simulink model "w31_v6"  (Simulink 7.9)
settings: Solver=FixedStepDiscrete  StartTime=0.0  StopTime=inf  FixedStep=0.01  RelTol=1e-3
undefined symbols (not defined in the file): DiscIntNeverNeededParam, magnitude
libraries: canmsglib x24, cansrvlib x22, simulink x12, iohwablib x5, legionoslib x3, ccpsrvlib x2, memsrvlib x1, tgttoollib x1, udssrvlib x1, wdgmlib x1
(part 2 of 5)

== system w31_v6/Logic_And_Algorithm/No_Signal_Emg_Judge ==
  Chassis_Signal : Inport
  Remote_Signal : Inport  Port=2
  Hardware_Signal : Inport  Port=3
  iECU_Signal : Inport  Port=4
  Bus Creator : BusCreator  Inputs=1
  Bus Creator1 : BusCreator  Inputs=1
  Bus Selector : BusSelector  OutputSignals=DBSF_Receive.DBSF_Status_NoRxMsg
  Bus Selector1 : BusSelector  OutputSignals=Remote_Analog.Remote_Analog_Status,Remote_IO.Remote_IO_Status
  Bus Selector2 : BusSelector  OutputSignals=Eme_Stop_Cmd,Front_Touch_Switch,Rear_Touch_Switch
  Bus Selector3 : BusSelector  OutputSignals=iECU_Status
  Logical Operator : Logic  Operator=OR  Inputs=6  AllPortsSameDT=off  OutDataTypeStr=boolean
  Logical Operator1 : Logic  Operator=OR  AllPortsSameDT=off  OutDataTypeStr=boolean
  No_Remote_CAN_Msg_Or_Emg_Button : Outport
  No_iECU_CAN_Msg_Or_Emg_Button : Outport  Port=2
  wires:
  Chassis_Signal/1 -> Bus Selector/1
  Remote_Signal/1 -> Bus Selector1/1
  Hardware_Signal/1 -> Bus Selector2/1
  iECU_Signal/1 -> Bus Selector3/1
  Bus Selector/1 -> Logical Operator/1  "<DBSF_Status_NoRxMsg>"
  Bus Selector1/1 -> Logical Operator/3  "<Remote_Analog_Status>"
  Bus Selector1/2 -> Logical Operator/4  "<Remote_IO_Status>"
  Logical Operator/1 -> Bus Creator/1, Logical Operator1/1  "No_Remote_CAN_Msg_Or_Emg_Button"
  Logical Operator1/1 -> Bus Creator1/1  "No_iECU_CAN_Msg_Or_Emg_Button"
  Bus Selector3/1 -> Logical Operator1/2  "<iECU_Status>"
  Bus Creator/1 -> No_Remote_CAN_Msg_Or_Emg_Button/1  "No_Remote_CAN_Msg_Or_Emg_Button"
  Bus Creator1/1 -> No_iECU_CAN_Msg_Or_Emg_Button/1
  Bus Selector2/1 -> Logical Operator/2  "<Eme_Stop_Cmd>"
  Bus Selector2/2 -> Logical Operator/5  "<Front_Touch_Switch>"
  Bus Selector2/3 -> Logical Operator/6  "<Rear_Touch_Switch>"

== system w31_v6/Logic_And_Algorithm/Remote_mode_with_control_0 ==
  note: 驱动控制算法，等待填充分布式控制算法
  Chassis_CAN_input : Inport
  Sensor_CAN_input : Inport  Port=2
  Remote_CAN_input : Inport  Port=3
  Hardware_input : Inport  Port=4
  No_Remote_CAN_Msg_Or_Emg_Button : Inport  Port=5
  Action Port : ActionPort  ActionType=case
  Brake_calculation : Subsystem
  Bus Creator : BusCreator
  Bus Creator1 : BusCreator  Inputs=6
  Bus Creator2 : BusCreator  Inputs=2
  Power_calculation : Subsystem
  Signal_Input : Subsystem
  Steering_calculation : Subsystem
  Power_cal_to_CANBus : Outport
  Steering_cal_to_CANBus : Outport  Port=2
  Brake_to_CANBus : Outport  Port=3
  wires:
  Bus Creator/1 -> Power_cal_to_CANBus/1
  Chassis_CAN_input/1 -> Signal_Input/1(Chassis_CAN_input)
  Sensor_CAN_input/1 -> Signal_Input/2(Sensor_CAN_input)
  Remote_CAN_input/1 -> Signal_Input/3(Remote_CAN_input)
  Hardware_input/1 -> Signal_Input/4(Hardware_input)
  Bus Creator1/1 -> Steering_cal_to_CANBus/1
  Steering_calculation/1(F_Steering_Angle) -> Bus Creator1/1
  Steering_calculation/2(R_Steering_Angle) -> Bus Creator1/2
  Steering_calculation/3(F_Steering_Work_Mode) -> Bus Creator1/3
  Steering_calculation/4(R_Steering_Work_Mode) -> Bus Creator1/4
  Steering_calculation/5(F_Steering_Angle_Rate) -> Bus Creator1/5
  Steering_calculation/6(R_Steering_Angle_Rate) -> Bus Creator1/6
  No_Remote_CAN_Msg_Or_Emg_Button/1 -> Signal_Input/5(No_Remote_CAN_Msg_Or_Emg_Button)
  Brake_calculation/1(Break_Req) -> Bus Creator2/1  "Break_Req"
  Brake_calculation/2(Remote_EPB_Req) -> Bus Creator2/2  "Remote_EPB_Req"
  Bus Creator2/1 -> Brake_to_CANBus/1
  Power_calculation/1(Power_FL) -> Bus Creator/1
  Power_calculation/2(Power_FR) -> Bus Creator/2
  Power_calculation/3(Power_RL) -> Bus Creator/3
  Power_calculation/4(Power_RR) -> Bus Creator/4

== system w31_v6/Logic_And_Algorithm/Remote_mode_with_control_2 ==
  note: 驱动控制算法，等待填充分布式控制算法
  Remote_CAN_input : Inport
  Hardware_input : Inport  Port=2
  No_Remote_CAN_Msg_Or_Emg_Button : Inport  Port=3
  Action Port : ActionPort  ActionType=case
  Brake_calculation : Subsystem
  Bus Creator : BusCreator
  Bus Creator1 : BusCreator  Inputs=6
  Bus Creator2 : BusCreator  Inputs=2
  Power_calculation : Subsystem
  Signal_Input : Subsystem
  Steering_calculation : Subsystem
  Steering_cal_to_CANBus : Outport
  Brake_to_CANBus : Outport  Port=2
  Power_cal_to_CANBus : Outport  Port=3
  wires:
  No_Remote_CAN_Msg_Or_Emg_Button/1 -> Signal_Input/3(No_Remote_CAN_Msg_Or_Emg_Button)
  Hardware_input/1 -> Signal_Input/2(Hardware_input)
  Remote_CAN_input/1 -> Signal_Input/1(Remote_CAN_input)
  Bus Creator2/1 -> Brake_to_CANBus/1
  Brake_calculation/2(Remote_EPB_Req) -> Bus Creator2/2  "Remote_EPB_Req"
  Brake_calculation/1(Break_Req) -> Bus Creator2/1  "Break_Req"
  Steering_calculation/6(R_Steering_Angle_Rate) -> Bus Creator1/6
  Steering_calculation/5(F_Steering_Angle_Rate) -> Bus Creator1/5
  Steering_calculation/4(R_Steering_Work_Mode) -> Bus Creator1/4
  Steering_calculation/3(F_Steering_Work_Mode) -> Bus Creator1/3
  Steering_calculation/2(R_Steering_Angle) -> Bus Creator1/2
  Steering_calculation/1(F_Steering_Angle) -> Bus Creator1/1
  Bus Creator1/1 -> Steering_cal_to_CANBus/1
  Bus Creator/1 -> Power_cal_to_CANBus/1
  Power_calculation/1(Power_FL) -> Bus Creator/1
  Power_calculation/2(Power_FR) -> Bus Creator/2
  Power_calculation/3(Power_RL) -> Bus Creator/3
  Power_calculation/4(Power_RR) -> Bus Creator/4

== system w31_v6/Logic_And_Algorithm/Slop_Cal ==
  IMU_Ax : Inport
  Trigonometric Function : Trigonometry  Operator=asin
  Slop : Outport
  wires:
  IMU_Ax/1 -> Trigonometric Function/1
  Trigonometric Function/1 -> Slop/1

== system w31_v6/Logic_And_Algorithm/drive_mode_judegment ==
  note: Remote请求为0，iECU请求为1的情况下，输出非0，进入自动驾驶状态，否则为遥控驾驶
  Remote_CANbus : Inport
  iECU_CANbus : Inport  Port=2
  Bus Selector : BusSelector  OutputSignals=Remote_IO.Remote_or_iECU_Mode_Switch,Remote_IO.Remote_Control_Speed_or_Torque
  Bus Selector1 : BusSelector  OutputSignals=iECU_Control_Flag
  Data Type Conversion3 : DataTypeConversion  OutDataTypeStr=uint8
  MATLAB Function : MATLAB Function  TreatAsAtomicUnit=on
  drive_mode : Outport
  wires:
  Remote_CANbus/1 -> Bus Selector/1
  iECU_CANbus/1 -> Bus Selector1/1
  Bus Selector/1 -> MATLAB Function/1(remote_or_iECU)  "<Remote_or_iECU_Mode_Switch>"
  Bus Selector/2 -> MATLAB Function/2(remote_speed_or_torque)  "<Remote_Control_Speed_or_Torque>"
  Bus Selector1/1 -> MATLAB Function/3(iECU_control_flag)  "<iECU_Control_Flag>"
  MATLAB Function/1(drive_mode) -> Data Type Conversion3/1
  Data Type Conversion3/1 -> drive_mode/1

== system w31_v6/Logic_And_Algorithm/iECU_mode_with_control ==
  note: 驱动控制算法，等待填充分布式控制算法
  Chassis_CAN_input : Inport
  Sensor_CAN_input : Inport  Port=2
  Remote_CAN_input : Inport  Port=3
  Hardware_input : Inport  Port=4
  iECU_CAN_input : Inport  Port=5
  No_iECU_CAN_Msg_Or_Emg_Button : Inport  Port=6
  Action Port : ActionPort  ActionType=default
  Brake_calculation : Subsystem
  Bus Creator : BusCreator  Inputs=2
  Bus Creator1 : BusCreator  Inputs=6
  Power_calculation : Subsystem
  Signal_Input : Subsystem
  Steering_calculation : Subsystem
  Power_cal_to_CANBus : Outport
  Steering_cal_to_CANBus : Outport  Port=2
  Brake_to_CANBus : Outport  Port=3
  wires:
  Chassis_CAN_input/1 -> Signal_Input/1(Chassis_CAN_input)
  Sensor_CAN_input/1 -> Signal_Input/2(Sensor_CAN_input)
  Remote_CAN_input/1 -> Signal_Input/3(Remote_CAN_input)
  Hardware_input/1 -> Signal_Input/4(Hardware_input)
  iECU_CAN_input/1 -> Signal_Input/5(iECU_CAN_input)
  Bus Creator/1 -> Power_cal_to_CANBus/1
  Power_calculation/2(Torque_to_Motor_CANBus) -> Bus Creator/2
  Bus Creator1/1 -> Steering_cal_to_CANBus/1
  Steering_calculation/1(F_Steering_Angle) -> Bus Creator1/1
  Steering_calculation/2(R_Steering_Angle) -> Bus Creator1/2
  Steering_calculation/3(F_Steering_Work_Mode) -> Bus Creator1/3
  Steering_calculation/4(R_Steering_Work_Mode) -> Bus Creator1/4
  Steering_calculation/5(F_Steering_Angle_Rate) -> Bus Creator1/5
  Steering_calculation/6(R_Steering_Angle_Rate) -> Bus Creator1/6
  Brake_calculation/1(Break_Req) -> Brake_to_CANBus/1  "Break_Req"
  No_iECU_CAN_Msg_Or_Emg_Button/1 -> Signal_Input/6(No_iECU_CAN_Msg_Or_Emg_Button)
  Power_calculation/1(Rotation_to_Motor_CANBus) -> Bus Creator/1

== system w31_v6/10ms_Signal_Output/SteerCAN_Out1/F ==
  Command_Angle : Inport
  Bitwise Operator : simulink/Logic and Bit Operations/Bitwise Operator  logicop=XOR  UseBitMask=off  NumInputPorts=7  BitMask=bin2dec('11011001')  BitMaskRealWorld=Stored Integer
  CAN Pack1 : canmsglib/CAN Pack  CANdbFile=E:\matlab_ws\2012_Matlab_Vcu\w_serial\w3\w32\dbc\w32_CAN1_500kbs_0421_v15.dbc  MsgList=VCU_EPSF_Control_Request  MsgName=VCU_EPSF_Control_Request  MsgIDType=Standard (11-bit identifier)  MsgIdentifier=1129  MsgLength=8  SignalInfo=High_VCU_Req_EPSF_Target_Angle$24$8$1$2$1$0$1$0$0$255$#Low_VCU_Req_EPSF_Target_Angle$32$8$1$2$1$0$1$0$0$255$#VCU_Control_EPSF_Reserved_1$8$8$1$2$1$0$1$0$0$255$#VCU_Control_EPSF_Reserved_2$16$8$1$2$1$0$1$0$0$255$#VCU_EPSF_CheckSum$56$8$1$2$1$0$1$0$0$255$#VCU_Request_EPSF_Angle_Calibrate$40$8$1$2$1$0$1$0$0$255$#VCU_Request_EPSF_Angle_Speed$48$8$1$2$1$0$1$0$20$250$#VCU_Request_EPSF_Control_Mode$0$8$1$2$1$0$1$0$0$255$#  NSignals=8  StartBits=str2num('[int32(24);int32(32);int32(8);int32(16);int32(56);int32(40);int32(48);int32(0)]')  SignalSizes=str2num('[int32(8);int32(8);int32(8);int32(8);int32(8);int32(8);int32(8);int32(8)]')  ByteOrders=str2num('[int32(1);int32(1);int32(1);int32(1);int32(1);int32(1);int32(1);int32(1)]')  DataTypes=str2num('[int32(2);int32(2);int32(2);int32(2);int32(2);int32(2);int32(2);int32(2)]')  MultiplexTypes=str2num('[int32(1);int32(1);int32(1);int32(1);int32(1);int32(1);int32(1);int32(1)]')  MultiplexValues=str2num('[double(0);double(0);double(0);double(0);double(0);double(0);double(0);double(0)]')  Factors=str2num('[double(1);double(1);double(1);double(1);double(1);double(1);double(1);double(1)]')  Offsets=str2num('[double(0);double(0);double(0);double(0);double(0);double(0);double(0);double(0)]')  Minimums=str2num('[double(0);double(0);double(0);double(0);double(0);double(0);double(20);double(0)]')  Maximums=str2num('[double(255);double(255);double(255);double(255);double(255);double(255);double(250);double(255)]')  Remote=off
      settings: DataFormat=CANdb specified signals
  CAN Transmit1 : cansrvlib/CAN Transmit  useModule=CAN1  messageID=hex2dec('469')  messageType=Standard (11-bit identifier)  msg_priority=255  messageID_Numeric=1129  ECU=V11P51_00E170701_01
  Subsystem : Subsystem
  eps_control_mode : Constant  Value=200  OutDataTypeStr=uint8  SampleTime=-1
  eps_reserve_1 : Constant  Value=0  OutDataTypeStr=uint8  SampleTime=-1
  eps_reserve_2 : Constant  Value=0  OutDataTypeStr=uint8  SampleTime=-1
  eps_reserve_3 : Constant  Value=32  OutDataTypeStr=uint8  SampleTime=-1
  eps_reserve_4 : Constant  Value=0  OutDataTypeStr=uint8  SampleTime=-1
  wires:
  CAN Pack1/1 -> CAN Transmit1/1
  Command_Angle/1 -> Subsystem/1(deserved_angle)
  eps_reserve_4/1 -> CAN Pack1/3, Bitwise Operator/2
  Subsystem/1(cmd_angle_high) -> CAN Pack1/1, Bitwise Operator/4
  Subsystem/2(cmd_angle_low) -> CAN Pack1/2, Bitwise Operator/5
  eps_reserve_1/1 -> CAN Pack1/4, Bitwise Operator/3
  eps_reserve_2/1 -> CAN Pack1/6, Bitwise Operator/6
  eps_control_mode/1 -> CAN Pack1/7, Bitwise Operator/7
  eps_reserve_3/1 -> CAN Pack1/8, Bitwise Operator/1
  Bitwise Operator/1 -> CAN Pack1/5

== system w31_v6/10ms_Signal_Output/SteerCAN_Out1/R ==
  Command_Angle : Inport
  Bitwise Operator : simulink/Logic and Bit Operations/Bitwise Operator  logicop=XOR  UseBitMask=off  NumInputPorts=7  BitMask=bin2dec('11011001')  BitMaskRealWorld=Stored Integer
  CAN Pack1 : canmsglib/CAN Pack  CANdbFile=E:\matlab_ws\2012_Matlab_Vcu\w_serial\w3\w32\dbc\w32_CAN1_500kbs_0421_v15.dbc  MsgList=VCU_EPSR_Control_Request  MsgName=VCU_EPSR_Control_Request  MsgIDType=Standard (11-bit identifier)  MsgIdentifier=257  MsgLength=8  SignalInfo=High_VCU_Req_EPSR_Target_Angle$24$8$1$2$1$0$1$0$0$255$#Low_VCU_Req_EPSR_Target_Angle$32$8$1$2$1$0$1$0$0$255$#VCU_Control_EPSR_Reserved_1$8$8$1$2$1$0$1$0$0$255$#VCU_Control_EPSR_Reserved_2$16$8$1$2$1$0$1$0$0$255$#VCU_EPSR_CheckSum$56$8$1$2$1$0$1$0$0$255$#VCU_Request_EPSR_Angle_Config$40$8$1$2$1$0$1$0$0$255$#VCU_Request_EPSR_Angle_Speed$48$8$1$2$1$0$1$0$20$250$#VCU_Request_EPSR_Control$0$8$1$2$1$0$1$0$0$255$#  NSignals=8  StartBits=str2num('[int32(24);int32(32);int32(8);int32(16);int32(56);int32(40);int32(48);int32(0)]')  SignalSizes=str2num('[int32(8);int32(8);int32(8);int32(8);int32(8);int32(8);int32(8);int32(8)]')  ByteOrders=str2num('[int32(1);int32(1);int32(1);int32(1);int32(1);int32(1);int32(1);int32(1)]')  DataTypes=str2num('[int32(2);int32(2);int32(2);int32(2);int32(2);int32(2);int32(2);int32(2)]')  MultiplexTypes=str2num('[int32(1);int32(1);int32(1);int32(1);int32(1);int32(1);int32(1);int32(1)]')  MultiplexValues=str2num('[double(0);double(0);double(0);double(0);double(0);double(0);double(0);double(0)]')  Factors=str2num('[double(1);double(1);double(1);double(1);double(1);double(1);double(1);double(1)]')  Offsets=str2num('[double(0);double(0);double(0);double(0);double(0);double(0);double(0);double(0)]')  Minimums=str2num('[double(0);double(0);double(0);double(0);double(0);double(0);double(20);double(0)]')  Maximums=str2num('[double(255);double(255);double(255);double(255);double(255);double(255);double(250);double(255)]')  Remote=off
      settings: DataFormat=CANdb specified signals
  CAN Transmit1 : cansrvlib/CAN Transmit  useModule=CAN1  messageID=hex2dec('101')  messageType=Standard (11-bit identifier)  msg_priority=255  messageID_Numeric=257  ECU=V11P51_00E170701_01
  Subsystem : Subsystem
  eps_control_mode : Constant  Value=200  OutDataTypeStr=uint8  SampleTime=-1
  eps_reserve_1 : Constant  Value=0  OutDataTypeStr=uint8  SampleTime=-1
  eps_reserve_2 : Constant  Value=0  OutDataTypeStr=uint8  SampleTime=-1
  eps_reserve_3 : Constant  Value=32  OutDataTypeStr=uint8  SampleTime=-1
  eps_reserve_4 : Constant  Value=0  OutDataTypeStr=uint8  SampleTime=-1
  wires:
  CAN Pack1/1 -> CAN Transmit1/1
  eps_reserve_4/1 -> CAN Pack1/3, Bitwise Operator/2
  Subsystem/1(cmd_angle_high) -> CAN Pack1/1, Bitwise Operator/4
  Subsystem/2(cmd_angle_low) -> CAN Pack1/2, Bitwise Operator/5
  eps_reserve_1/1 -> CAN Pack1/4, Bitwise Operator/3
  eps_reserve_2/1 -> CAN Pack1/6, Bitwise Operator/6
  eps_control_mode/1 -> CAN Pack1/7, Bitwise Operator/7
  eps_reserve_3/1 -> CAN Pack1/8, Bitwise Operator/1
  Bitwise Operator/1 -> CAN Pack1/5
  Command_Angle/1 -> Subsystem/1(deserved_angle)

== system w31_v6/CAN_Receive_10ms/BMS_CAN/BMS ==
  msg : Inport
  Function : TriggerPort  TriggerType=function-call  PortDimensions=1
  Constant : Constant  OutDataTypeStr=uint8  SampleTime=-1
  Data Type Conversion1 : DataTypeConversion  OutDataTypeStr=uint8
  Data Type Conversion3 : DataTypeConversion  OutDataTypeStr=uint8
  Data Type Conversion4 : DataTypeConversion  OutDataTypeStr=uint8
  Memory : Memory  InheritSampleTime=on
  Remote_control_Io : canmsglib/CAN Unpack  CANdbFile=E:\matlab_ws\2012_Matlab_Vcu\w_serial\w3\w32\dbc\w32_CAN2_250kbs_0309_v5.dbc  MsgList=BMS_Status_1  MsgName=BMS_Status_1  MsgIDType=Extended (29-bit identifier)  MsgIdentifier=419375348  MsgLength=8  SignalInfo=Batter_Ready_Status$3$1$1$2$1$0$1$0$0$1$#Battery_Discharge_Current$16$16$1$2$1$0$1.000000e-01$-500$-500$500$#Battery_Falt_Code$56$8$1$2$1$0$1$0$0$255$#Battery_Fault_Grade$48$8$1$2$1$0$1$0$0$3$#Battery_Heating_Relay_Status$6$1$1$2$1$0$1$0$0$1$#Battery_Voltage$32$16$1$2$1$0$1.000000e-01$0$0$1000$#Charge_Relay_Status$5$1$1$2$1$0$1$0$0$1$#Charge_Status$1$1$1$2$1$0$1$0$0$1$#Charge_Wire_Connection_Status$0$1$1$2$1$0$1$0$0$1$#Discharge_Relay_Status$4$1$1$2$1$0$1$0$0$1$#Loss_of_Capacity_Status$2$1$1$2$1$0$1$0$0$1$#Precharge_Realy_Status$7$1$1$2$1$0$1$0$0$1$#SOC$8$8$1$2$1$0$1$0$0$255$#  NSignals=13  IDPort=off  TimestampPort=off  ErrorPort=off  RemotePort=off  LengthPort=off  StatusPort=off  StartBits=str2num('[int32(3);int32(16);int32(56);int32(48);int32(6);int32(32);int32(5);int32(1);int32(0);int32(4);int32(2);int32(7);int32(8)]')  SignalSizes=str2num('[int32(1);int32(16);int32(8);int32(8);int32(1);int32(16);int32(1);int32(1);int32(1);int32(1);int32(1);int32(1);int32(8)]')  ByteOrders=str2num('[int32(1);int32(1);int32(1);int32(1);int32(1);int32(1);int32(1);int32(1);int32(1);int32(1);int32(1);int32(1);int32(1)]')  DataTypes=str2num('[int32(2);int32(2);int32(2);int32(2);int32(2);int32(2);int32(2);int32(2);int32(2);int32(2);int32(2);int32(2);int32(2)]')  MultiplexTypes=str2num('[int32(1);int32(1);int32(1);int32(1);int32(1);int32(1);int32(1);int32(1);int32(1);int32(1);int32(1);int32(1);int32(1)]')  MultiplexValues=str2num('[double(0);double(0);double(0);double(0);double(0);double(0);double(0);double(0);double(0);double(0);double(0);double(0);double(0)]')  Factors=str2num('[double(1);double(1.000000e-01);double(1);double(1);double(1);double(1.000000e-01);double(1);double(1);double(1);double(1);double(1);double(1);double(1)]')  Offsets=str2num('[double(0);double(-500);double(0);double(0);double(0);double(0);double(0);double(0);double(0);double(0);double(0);double(0);double(0)]')  Minimums=str2num('[double(0);double(-500);double(0);double(0);double(0);double(0);double(0);double(0);double(0);double(0);double(0);double(0);double(0)]')  Maximums=str2num('[double(1);double(500);double(255);double(3);double(1);double(1000);double(1);double(1);double(1);double(1);double(1);double(1);double(255)]')
      settings: DataFormat=CANdb specified signals
  Sum : Sum  Inputs=|++  OutDataTypeStr=uint8
  BatteryFaultGrade : Outport
  DischargeRelayStatus : Outport  Port=2
  BMS_Loss_of_Capacity : Outport  Port=3
  BMS_Stutas : Outport  Port=4
  wires:
  Memory/1 -> Sum/2
  Sum/1 -> Memory/1, BMS_Stutas/1
  Constant/1 -> Sum/1
  msg/1 -> Remote_control_Io/1
  Remote_control_Io/4 -> Data Type Conversion3/1
  Remote_control_Io/10 -> Data Type Conversion4/1
  Data Type Conversion3/1 -> BatteryFaultGrade/1  "BatteryFaultGrade"
  Data Type Conversion4/1 -> DischargeRelayStatus/1  "DischargeRelayStatus"
  Remote_control_Io/11 -> Data Type Conversion1/1
  Data Type Conversion1/1 -> BMS_Loss_of_Capacity/1  "BMS_Loss_of_Capacity"

== system w31_v6/CAN_Receive_10ms/BMS_CAN/shake_situation1 ==
  note: 输出1表示信号丢失
      | 输出0表示一切正常
  RxMsgCnt : Inport
  NoRxMsgCntMax : Inport  Port=2
  Chart : Stateflow chart  TreatAsAtomicUnit=on
  Relational Operator1 : RelationalOperator  Operator=~=  OutDataTypeStr=boolean
  Terminator : Terminator
  Unit Delay1 : UnitDelay  SampleTime=-1
  NoRxMsgComfirm : Outport
  wires:
  NoRxMsgCntMax/1 -> Chart/2(NoRxMsgCntMax)
  Unit Delay1/1 -> Relational Operator1/1
  RxMsgCnt/1 -> Relational Operator1/2, Unit Delay1/1
  Relational Operator1/1 -> Chart/1(RxMsg)
  Chart/1(NoRxMsgComfirm) -> NoRxMsgComfirm/1
  Chart/2(NoRxMsgCnt) -> Terminator/1

== system w31_v6/CAN_Receive_10ms/Chassis_CAN/DBSF ==
  msg : Inport
  Function : TriggerPort  TriggerType=function-call  PortDimensions=1
  Constant : Constant  OutDataTypeStr=uint8  SampleTime=-1
  DBSR : canmsglib/CAN Unpack  CANdbFile=D:\W31_workspace\w31_CAN1_500kbs_0618_v5.1.dbc  MsgList=DBSF_Status  MsgName=DBSF_Status  MsgIDType=Standard (11-bit identifier)  MsgIdentifier=322  MsgLength=8  SignalInfo=DBSF_Fault_Code$32$8$1$2$1$0$1$0$0$255$#DBSF_HP_pressure$16$16$1$2$1$0$1.000000e-02$0$0$8$#DBSF_Reserved_1$2$14$1$2$1$0$1$0$0$500$#DBSF_Reserved_2$40$24$1$2$1$0$1$0$0$500$#DBSF_System_Status$0$2$1$2$1$0$1$0$0$3$#  NSignals=5  IDPort=off  TimestampPort=off  ErrorPort=off  RemotePort=off  LengthPort=off  StatusPort=off  StartBits=str2num('[int32(32);int32(16);int32(2);int32(40);int32(0)]')  SignalSizes=str2num('[int32(8);int32(16);int32(14);int32(24);int32(2)]')  ByteOrders=str2num('[int32(1);int32(1);int32(1);int32(1);int32(1)]')  DataTypes=str2num('[int32(2);int32(2);int32(2);int32(2);int32(2)]')  MultiplexTypes=str2num('[int32(1);int32(1);int32(1);int32(1);int32(1)]')  MultiplexValues=str2num('[double(0);double(0);double(0);double(0);double(0)]')  Factors=str2num('[double(1);double(1.000000e-02);double(1);double(1);double(1)]')  Offsets=str2num('[double(0);double(0);double(0);double(0);double(0)]')  Minimums=str2num('[double(0);double(0);double(0);double(0);double(0)]')  Maximums=str2num('[double(255);double(8);double(500);double(500);double(3)]')
      settings: DataFormat=CANdb specified signals
  Memory : Memory  InheritSampleTime=on
  Sum : Sum  Inputs=|++  OutDataTypeStr=uint8
  Terminator{1..2,4..5} (4 alike) : Terminator
  DBSF_HP_Pressure : Outport
  DBSF_Status : Outport  Port=2
  wires:
  Memory/1 -> Sum/2
  Sum/1 -> Memory/1, DBSF_Status/1
  Constant/1 -> Sum/1
  msg/1 -> DBSR/1
  DBSR/3 -> Terminator2/1
  DBSR/5 -> Terminator4/1
  DBSR/4 -> Terminator5/1
  DBSR/1 -> Terminator1/1
  DBSR/2 -> DBSF_HP_Pressure/1

== system w31_v6/CAN_Receive_10ms/Chassis_CAN/DBSF_NoMsg ==
  note: 输出1表示信号丢失
      | 输出0表示一切正常
  RxMsgCnt : Inport
  NoRxMsgCntMax : Inport  Port=2
  Chart : Stateflow chart  TreatAsAtomicUnit=on
  Relational Operator1 : RelationalOperator  Operator=~=  OutDataTypeStr=boolean
  Terminator : Terminator
  Unit Delay1 : UnitDelay  SampleTime=-1
  NoRxMsgComfirm : Outport
  wires:
  Chart/2(NoRxMsgCnt) -> Terminator/1
  Chart/1(NoRxMsgComfirm) -> NoRxMsgComfirm/1
  Relational Operator1/1 -> Chart/1(RxMsg)
  RxMsgCnt/1 -> Unit Delay1/1, Relational Operator1/2
  Unit Delay1/1 -> Relational Operator1/1
  NoRxMsgCntMax/1 -> Chart/2(NoRxMsgCntMax)

== system w31_v6/CAN_Receive_10ms/Chassis_CAN/EPSF ==
  note: 目前这个DBC没有更新为W31-0618-v5.1
      | 申 20200619
  msg : Inport
  Function : TriggerPort  TriggerType=function-call  PortDimensions=1
  Constant : Constant  OutDataTypeStr=uint8  SampleTime=-1
  Constant1 : Constant  Value=256  OutDataTypeStr=uint16  SampleTime=-1
  Constant2 : Constant  Value=1024  OutDataTypeStr=uint16  SampleTime=-1
  DBSR : canmsglib/CAN Unpack  CANdbFile=E:\matlab_ws\2012_Matlab_Vcu\w_serial\w3\w32\dbc\w32_CAN1_500kbs_0322_v7.dbc  MsgList=EPSF_Status  MsgName=EPSF_Status  MsgIDType=Standard (11-bit identifier)  MsgIdentifier=1025  MsgLength=8  SignalInfo=EPSF_Angle_In_Middle_Calib$40$8$1$2$1$0$1$0$0$255$#EPSF_Check_Sum$56$8$1$2$1$0$1$0$0$255$#EPSF_Reserved1$16$8$1$1$1$0$1$0$0$255$#EPSF_Reserved2$48$8$1$2$1$0$1$0$0$255$#EPSF_Steering_Wheel_Torque_Value$8$8$1$2$1$0$1.000000e-01$-1.280000e+01$-1.270000e+01$1.260000e+01$#EPSF_Work_Mode_Status$0$8$1$2$1$0$1$0$0$255$#High_EPSF_Angle$24$8$1$2$1$0$1$0$0$255$#Low_EPSF_Angle$32$8$1$2$1$0$1$0$0$255$#  NSignals=8  IDPort=off  TimestampPort=off  ErrorPort=off  RemotePort=off  LengthPort=off  StatusPort=off  StartBits=str2num('[int32(40);int32(56);int32(16);int32(48);int32(8);int32(0);int32(24);int32(32)]')  SignalSizes=str2num('[int32(8);int32(8);int32(8);int32(8);int32(8);int32(8);int32(8);int32(8)]')  ByteOrders=str2num('[int32(1);int32(1);int32(1);int32(1);int32(1);int32(1);int32(1);int32(1)]')  DataTypes=str2num('[int32(2);int32(2);int32(1);int32(2);int32(2);int32(2);int32(2);int32(2)]')  MultiplexTypes=str2num('[int32(1);int32(1);int32(1);int32(1);int32(1);int32(1);int32(1);int32(1)]')  MultiplexValues=str2num('[double(0);double(0);double(0);double(0);double(0);double(0);double(0);double(0)]')  Factors=str2num('[double(1);double(1);double(1);double(1);double(1.000000e-01);double(1);double(1);double(1)]')  Offsets=str2num('[double(0);double(0);double(0);double(0);double(-1.280000e+01);double(0);double(0);double(0)]')  Minimums=str2num('[double(0);double(0);double(0);double(0);double(-1.270000e+01);double(0);double(0);double(0)]')  Maximums=str2num('[double(255);double(255);double(255);double(255);double(1.260000e+01);double(255);double(255);double(255)]')
      settings: DataFormat=CANdb specified signals
  Gain : Gain  Gain=1/15.5  OutDataTypeStr=double
  Memory : Memory  InheritSampleTime=on
  Product : Product  RndMeth=Zero
  Sum : Sum  Inputs=|++  OutDataTypeStr=uint8
  Sum1 : Sum  Inputs=|++-  OutDataTypeStr=int16
  Terminator{1..6} (6 alike) : Terminator
  F_Tire_Angle_Feedback : Outport
  EPSF_Status : Outport  Port=2
  wires:
  Memory/1 -> Sum/2
  Sum/1 -> Memory/1, EPSF_Status/1
  Constant/1 -> Sum/1
  msg/1 -> DBSR/1
  DBSR/1 -> Terminator1/1
  DBSR/2 -> Terminator2/1
  DBSR/3 -> Terminator5/1
  DBSR/4 -> Terminator4/1
  DBSR/5 -> Terminator3/1
  DBSR/6 -> Terminator6/1
  DBSR/7 -> Product/1
  Constant1/1 -> Product/2
  Product/1 -> Sum1/1
  DBSR/8 -> Sum1/2
  Constant2/1 -> Sum1/3
  Sum1/1 -> Gain/1
  Gain/1 -> F_Tire_Angle_Feedback/1

== system w31_v6/CAN_Receive_10ms/Chassis_CAN/EPSF_NoMsg ==
  note: 输出1表示信号丢失
      | 输出0表示一切正常
  RxMsgCnt : Inport
  NoRxMsgCntMax : Inport  Port=2
  Chart : Stateflow chart  TreatAsAtomicUnit=on
  Relational Operator1 : RelationalOperator  Operator=~=  OutDataTypeStr=boolean
  Terminator : Terminator
  Unit Delay1 : UnitDelay  SampleTime=-1
  NoRxMsgComfirm : Outport
  wires:
  Chart/2(NoRxMsgCnt) -> Terminator/1
  Chart/1(NoRxMsgComfirm) -> NoRxMsgComfirm/1
  Relational Operator1/1 -> Chart/1(RxMsg)
  RxMsgCnt/1 -> Unit Delay1/1, Relational Operator1/2
  Unit Delay1/1 -> Relational Operator1/1
  NoRxMsgCntMax/1 -> Chart/2(NoRxMsgCntMax)

== system w31_v6/CAN_Receive_10ms/Chassis_CAN/EPSR ==
  note: 目前这个DBC没有更新为W31-0618-v5.1
      | 申 20200619
  msg : Inport
  Function : TriggerPort  TriggerType=function-call  PortDimensions=1
  Constant : Constant  OutDataTypeStr=uint8  SampleTime=-1
  Constant1 : Constant  Value=256  OutDataTypeStr=uint16  SampleTime=-1
  Constant2 : Constant  Value=1024  OutDataTypeStr=uint16  SampleTime=-1
  DBSR : canmsglib/CAN Unpack  CANdbFile=E:\matlab_ws\2012_Matlab_Vcu\w_serial\w3\w32\dbc\w32_CAN1_500kbs_0322_v7.dbc  MsgList=EPSR_Status  MsgName=EPSR_Status  MsgIDType=Standard (11-bit identifier)  MsgIdentifier=273  MsgLength=8  SignalInfo=EPSR_Angle_In_Middle_Calib$40$8$1$2$1$0$1$0$0$255$#EPSR_Check_Sum$56$8$1$2$1$0$1$0$0$255$#EPSR_Reserved1$16$8$1$2$1$0$1$0$0$255$#EPSR_Reserved2$48$8$1$2$1$0$1$0$0$255$#EPSR_Steering_Wheel_Torque_Value$8$8$1$2$1$0$1.000000e-01$-1.280000e+01$-1.270000e+01$1.260000e+01$#EPSR_Work_Mode_Status$0$8$1$2$1$0$1$0$0$255$#High_EPSR_Angle$24$8$1$2$1$0$1$0$0$255$#Low_EPSR_Angle$32$8$1$2$1$0$1$0$0$255$#  NSignals=8  IDPort=off  TimestampPort=off  ErrorPort=off  RemotePort=off  LengthPort=off  StatusPort=off  StartBits=str2num('[int32(40);int32(56);int32(16);int32(48);int32(8);int32(0);int32(24);int32(32)]')  SignalSizes=str2num('[int32(8);int32(8);int32(8);int32(8);int32(8);int32(8);int32(8);int32(8)]')  ByteOrders=str2num('[int32(1);int32(1);int32(1);int32(1);int32(1);int32(1);int32(1);int32(1)]')  DataTypes=str2num('[int32(2);int32(2);int32(2);int32(2);int32(2);int32(2);int32(2);int32(2)]')  MultiplexTypes=str2num('[int32(1);int32(1);int32(1);int32(1);int32(1);int32(1);int32(1);int32(1)]')  MultiplexValues=str2num('[double(0);double(0);double(0);double(0);double(0);double(0);double(0);double(0)]')  Factors=str2num('[double(1);double(1);double(1);double(1);double(1.000000e-01);double(1);double(1);double(1)]')  Offsets=str2num('[double(0);double(0);double(0);double(0);double(-1.280000e+01);double(0);double(0);double(0)]')  Minimums=str2num('[double(0);double(0);double(0);double(0);double(-1.270000e+01);double(0);double(0);double(0)]')  Maximums=str2num('[double(255);double(255);double(255);double(255);double(1.260000e+01);double(255);double(255);double(255)]')
      settings: DataFormat=CANdb specified signals
  Gain : Gain  Gain=-1/15.5  OutDataTypeStr=double
  Memory : Memory  InheritSampleTime=on
  Product : Product  RndMeth=Zero
  Sum : Sum  Inputs=|++  OutDataTypeStr=uint8
  Sum1 : Sum  Inputs=|++-  OutDataTypeStr=int16
  Terminator{1..6} (6 alike) : Terminator
  R_Tire_Angle_Feedback : Outport
  EPSR_Status : Outport  Port=2
  wires:
  Memory/1 -> Sum/2
  Sum/1 -> Memory/1, EPSR_Status/1
  Constant/1 -> Sum/1
  msg/1 -> DBSR/1
  DBSR/1 -> Terminator1/1
  DBSR/2 -> Terminator2/1
  DBSR/3 -> Terminator5/1
  DBSR/4 -> Terminator4/1
  DBSR/5 -> Terminator3/1
  DBSR/6 -> Terminator6/1
  DBSR/7 -> Product/1
  Constant1/1 -> Product/2
  Product/1 -> Sum1/1
  DBSR/8 -> Sum1/2
  Constant2/1 -> Sum1/3
  Sum1/1 -> Gain/1
  Gain/1 -> R_Tire_Angle_Feedback/1

== system w31_v6/CAN_Receive_10ms/Chassis_CAN/EPSR_NoMsg ==
  note: 输出1表示信号丢失
      | 输出0表示一切正常
  RxMsgCnt : Inport
  NoRxMsgCntMax : Inport  Port=2
  Chart : Stateflow chart  TreatAsAtomicUnit=on
  Relational Operator1 : RelationalOperator  Operator=~=  OutDataTypeStr=boolean
  Terminator : Terminator
  Unit Delay1 : UnitDelay  SampleTime=-1
  NoRxMsgComfirm : Outport
  wires:
  Chart/2(NoRxMsgCnt) -> Terminator/1
  Chart/1(NoRxMsgComfirm) -> NoRxMsgComfirm/1
  Relational Operator1/1 -> Chart/1(RxMsg)
  RxMsgCnt/1 -> Unit Delay1/1, Relational Operator1/2
  Unit Delay1/1 -> Relational Operator1/1
  NoRxMsgCntMax/1 -> Chart/2(NoRxMsgCntMax)

== system w31_v6/CAN_Receive_10ms/Chassis_CAN/FL_Motor ==
  msg : Inport
  Function : TriggerPort  TriggerType=function-call  PortDimensions=1
  Constant : Constant  OutDataTypeStr=uint8  SampleTime=-1
  Memory : Memory  InheritSampleTime=on
  Remote_control_Io : canmsglib/CAN Unpack  CANdbFile=D:\W31_workspace\w31_CAN1_500kbs_0618_v5.1.dbc  MsgList=MCUFL_Torque_Feedback  MsgName=MCUFL_Torque_Feedback  MsgIDType=Standard (11-bit identifier)  MsgIdentifier=16  MsgLength=8  SignalInfo=FL_CURRENT$36$12$1$2$1$0$1$-500$-500$500$#FL_ERRORCODE$56$8$1$2$1$0$1$0$0$255$#FL_MOTORTEMP$48$8$1$2$1$0$1$-50$-50$205$#FL_SPEED$2$18$1$2$1$0$1.000000e-01$-10000$-10000$10000$#FL_Shift$0$2$1$2$1$0$1$0$0$3$#FL_TORQUE$20$16$1$2$1$0$1.000000e-01$-1000$-1000$1000$#  NSignals=6  IDPort=off  TimestampPort=off  ErrorPort=off  RemotePort=off  LengthPort=off  StatusPort=off  StartBits=str2num('[int32(36);int32(56);int32(48);int32(2);int32(0);int32(20)]')  SignalSizes=str2num('[int32(12);int32(8);int32(8);int32(18);int32(2);int32(16)]')  ByteOrders=str2num('[int32(1);int32(1);int32(1);int32(1);int32(1);int32(1)]')  DataTypes=str2num('[int32(2);int32(2);int32(2);int32(2);int32(2);int32(2)]')  MultiplexTypes=str2num('[int32(1);int32(1);int32(1);int32(1);int32(1);int32(1)]')  MultiplexValues=str2num('[double(0);double(0);double(0);double(0);double(0);double(0)]')  Factors=str2num('[double(1);double(1);double(1);double(1.000000e-01);double(1);double(1.000000e-01)]')  Offsets=str2num('[double(-500);double(0);double(-50);double(-10000);double(0);double(-1000)]')  Minimums=str2num('[double(-500);double(0);double(-50);double(-10000);double(0);double(-1000)]')  Maximums=str2num('[double(500);double(255);double(205);double(10000);double(3);double(1000)]')
      settings: DataFormat=CANdb specified signals
  Sum : Sum  Inputs=|++  OutDataTypeStr=uint8
  Terminator{1..4} (4 alike) : Terminator
  FL_RPM_Feedback : Outport
  FL_Torque_Feedback : Outport  Port=2
  FL_MotorStatus : Outport  Port=3
  wires:
  Memory/1 -> Sum/2
  Sum/1 -> Memory/1, FL_MotorStatus/1
  Constant/1 -> Sum/1
  msg/1 -> Remote_control_Io/1
  Remote_control_Io/1 -> Terminator3/1
  Remote_control_Io/2 -> Terminator1/1
  Remote_control_Io/3 -> Terminator2/1
  Remote_control_Io/4 -> FL_RPM_Feedback/1
  Remote_control_Io/5 -> Terminator4/1
  Remote_control_Io/6 -> FL_Torque_Feedback/1

== system w31_v6/CAN_Receive_10ms/Chassis_CAN/FL_Motor_NoMsg ==
  note: 输出1表示信号丢失
      | 输出0表示一切正常
  RxMsgCnt : Inport
  NoRxMsgCntMax : Inport  Port=2
  Chart : Stateflow chart  TreatAsAtomicUnit=on
  Relational Operator1 : RelationalOperator  Operator=~=  OutDataTypeStr=boolean
  Terminator : Terminator
  Unit Delay1 : UnitDelay  SampleTime=-1
  NoRxMsgComfirm : Outport
  wires:
  NoRxMsgCntMax/1 -> Chart/2(NoRxMsgCntMax)
  Unit Delay1/1 -> Relational Operator1/1
  RxMsgCnt/1 -> Relational Operator1/2, Unit Delay1/1
  Relational Operator1/1 -> Chart/1(RxMsg)
  Chart/1(NoRxMsgComfirm) -> NoRxMsgComfirm/1
  Chart/2(NoRxMsgCnt) -> Terminator/1

== system w31_v6/CAN_Receive_10ms/Chassis_CAN/FR_Motor ==
  msg : Inport
  Function : TriggerPort  TriggerType=function-call  PortDimensions=1
  Constant : Constant  OutDataTypeStr=uint8  SampleTime=-1
  Memory : Memory  InheritSampleTime=on
  Remote_control_Io : canmsglib/CAN Unpack  CANdbFile=D:\W31_workspace\w31_CAN1_500kbs_0618_v5.1.dbc  MsgList=MCUFR_Torque_Feedback  MsgName=MCUFR_Torque_Feedback  MsgIDType=Standard (11-bit identifier)  MsgIdentifier=32  MsgLength=8  SignalInfo=FR_CURRENT$36$12$1$2$1$0$1$-500$-500$500$#FR_ERRORCODE$56$8$1$2$1$0$1$0$0$255$#FR_MOTORTEMP$48$8$1$2$1$0$1$-50$-50$205$#FR_SPEED$2$18$1$2$1$0$1.000000e-01$-10000$-10000$10000$#FR_Shift$0$2$1$2$1$0$1$0$0$3$#FR_TORQUE$20$16$1$2$1$0$1.000000e-01$-1000$-1000$1000$#  NSignals=6  IDPort=off  TimestampPort=off  ErrorPort=off  RemotePort=off  LengthPort=off  StatusPort=off  StartBits=str2num('[int32(36);int32(56);int32(48);int32(2);int32(0);int32(20)]')  SignalSizes=str2num('[int32(12);int32(8);int32(8);int32(18);int32(2);int32(16)]')  ByteOrders=str2num('[int32(1);int32(1);int32(1);int32(1);int32(1);int32(1)]')  DataTypes=str2num('[int32(2);int32(2);int32(2);int32(2);int32(2);int32(2)]')  MultiplexTypes=str2num('[int32(1);int32(1);int32(1);int32(1);int32(1);int32(1)]')  MultiplexValues=str2num('[double(0);double(0);double(0);double(0);double(0);double(0)]')  Factors=str2num('[double(1);double(1);double(1);double(1.000000e-01);double(1);double(1.000000e-01)]')  Offsets=str2num('[double(-500);double(0);double(-50);double(-10000);double(0);double(-1000)]')  Minimums=str2num('[double(-500);double(0);double(-50);double(-10000);double(0);double(-1000)]')  Maximums=str2num('[double(500);double(255);double(205);double(10000);double(3);double(1000)]')
      settings: DataFormat=CANdb specified signals
  Sum : Sum  Inputs=|++  OutDataTypeStr=uint8
  Terminator{1..4} (4 alike) : Terminator
  FR_RPM_Feedback : Outport
  FR_Torque_Feedback : Outport  Port=2
  FR_MotorStatus : Outport  Port=3
  wires:
  Memory/1 -> Sum/2
  Sum/1 -> Memory/1, FR_MotorStatus/1
  Constant/1 -> Sum/1
  msg/1 -> Remote_control_Io/1
  Remote_control_Io/1 -> Terminator3/1
  Remote_control_Io/2 -> Terminator1/1
  Remote_control_Io/3 -> Terminator2/1
  Remote_control_Io/4 -> FR_RPM_Feedback/1
  Remote_control_Io/5 -> Terminator4/1
  Remote_control_Io/6 -> FR_Torque_Feedback/1

== system w31_v6/CAN_Receive_10ms/Chassis_CAN/FR_Motor_NoMsg ==
  note: 输出1表示信号丢失
      | 输出0表示一切正常
  RxMsgCnt : Inport
  NoRxMsgCntMax : Inport  Port=2
  Chart : Stateflow chart  TreatAsAtomicUnit=on
  Relational Operator1 : RelationalOperator  Operator=~=  OutDataTypeStr=boolean
  Terminator : Terminator
  Unit Delay1 : UnitDelay  SampleTime=-1
  NoRxMsgComfirm : Outport
  wires:
  NoRxMsgCntMax/1 -> Chart/2(NoRxMsgCntMax)
  Unit Delay1/1 -> Relational Operator1/1
  RxMsgCnt/1 -> Relational Operator1/2, Unit Delay1/1
  Relational Operator1/1 -> Chart/1(RxMsg)
  Chart/1(NoRxMsgComfirm) -> NoRxMsgComfirm/1
  Chart/2(NoRxMsgCnt) -> Terminator/1

== system w31_v6/CAN_Receive_10ms/Chassis_CAN/RL_Motor ==
  msg : Inport
  Function : TriggerPort  TriggerType=function-call  PortDimensions=1
  Constant : Constant  OutDataTypeStr=uint8  SampleTime=-1
  MCU_RL : canmsglib/CAN Unpack  CANdbFile=D:\W31_workspace\w31_CAN1_500kbs_0618_v5.1.dbc  MsgList=MCURL_Torque_Feedback  MsgName=MCURL_Torque_Feedback  MsgIDType=Standard (11-bit identifier)  MsgIdentifier=48  MsgLength=8  SignalInfo=RL_CURRENT$36$12$1$2$1$0$1$-500$-500$500$#RL_ERRORCODE$56$8$1$2$1$0$1$0$0$255$#RL_MOTORTEMP$48$8$1$2$1$0$1$-50$-50$205$#RL_SPEED$2$18$1$2$1$0$1.000000e-01$-10000$-10000$10000$#RL_Shift$0$2$1$2$1$0$1$0$0$3$#RL_TORQUE$20$16$1$2$1$0$1.000000e-01$-1000$-1000$1000$#  NSignals=6  IDPort=off  TimestampPort=off  ErrorPort=off  RemotePort=off  LengthPort=off  StatusPort=off  StartBits=str2num('[int32(36);int32(56);int32(48);int32(2);int32(0);int32(20)]')  SignalSizes=str2num('[int32(12);int32(8);int32(8);int32(18);int32(2);int32(16)]')  ByteOrders=str2num('[int32(1);int32(1);int32(1);int32(1);int32(1);int32(1)]')  DataTypes=str2num('[int32(2);int32(2);int32(2);int32(2);int32(2);int32(2)]')  MultiplexTypes=str2num('[int32(1);int32(1);int32(1);int32(1);int32(1);int32(1)]')  MultiplexValues=str2num('[double(0);double(0);double(0);double(0);double(0);double(0)]')  Factors=str2num('[double(1);double(1);double(1);double(1.000000e-01);double(1);double(1.000000e-01)]')  Offsets=str2num('[double(-500);double(0);double(-50);double(-10000);double(0);double(-1000)]')  Minimums=str2num('[double(-500);double(0);double(-50);double(-10000);double(0);double(-1000)]')  Maximums=str2num('[double(500);double(255);double(205);double(10000);double(3);double(1000)]')
      settings: DataFormat=CANdb specified signals
  Memory : Memory  InheritSampleTime=on
  Sum : Sum  Inputs=|++  OutDataTypeStr=uint8
  Terminator{1..4} (4 alike) : Terminator
  RL_RPM_Feedback : Outport
  RL_Torque_Feedback : Outport  Port=2
  RL_MotorStatus : Outport  Port=3
  wires:
  Memory/1 -> Sum/2
  Sum/1 -> Memory/1, RL_MotorStatus/1
  Constant/1 -> Sum/1
  msg/1 -> MCU_RL/1
  MCU_RL/1 -> Terminator3/1
  MCU_RL/2 -> Terminator1/1
  MCU_RL/3 -> Terminator2/1
  MCU_RL/4 -> RL_RPM_Feedback/1
  MCU_RL/5 -> Terminator4/1
  MCU_RL/6 -> RL_Torque_Feedback/1

== system w31_v6/CAN_Receive_10ms/Chassis_CAN/RL_Motor_NoMsg ==
  note: 输出1表示信号丢失
      | 输出0表示一切正常
  RxMsgCnt : Inport
  NoRxMsgCntMax : Inport  Port=2
  Chart : Stateflow chart  TreatAsAtomicUnit=on
  Relational Operator1 : RelationalOperator  Operator=~=  OutDataTypeStr=boolean
  Terminator : Terminator
  Unit Delay1 : UnitDelay  SampleTime=-1
  NoRxMsgComfirm : Outport
  wires:
  NoRxMsgCntMax/1 -> Chart/2(NoRxMsgCntMax)
  Unit Delay1/1 -> Relational Operator1/1
  RxMsgCnt/1 -> Relational Operator1/2, Unit Delay1/1
  Relational Operator1/1 -> Chart/1(RxMsg)
  Chart/1(NoRxMsgComfirm) -> NoRxMsgComfirm/1
  Chart/2(NoRxMsgCnt) -> Terminator/1

== system w31_v6/CAN_Receive_10ms/Chassis_CAN/RR_Motor ==
  msg : Inport
  Function : TriggerPort  TriggerType=function-call  PortDimensions=1
  Constant : Constant  OutDataTypeStr=uint8  SampleTime=-1
  MCU_RR : canmsglib/CAN Unpack  CANdbFile=D:\W31_workspace\w31_CAN1_500kbs_0618_v5.1.dbc  MsgList=MCURR_Torque_Feedback  MsgName=MCURR_Torque_Feedback  MsgIDType=Standard (11-bit identifier)  MsgIdentifier=64  MsgLength=8  SignalInfo=RR_CURRENT$36$12$1$2$1$0$1$-500$-500$500$#RR_ERRORCODE$56$8$1$2$1$0$1$0$0$255$#RR_MOTORTEMP$48$8$1$2$1$0$1$-50$-50$205$#RR_SPEED$2$18$1$2$1$0$1.000000e-01$-10000$-10000$10000$#RR_Shift$0$2$1$2$1$0$1$0$0$3$#RR_TORQUE$20$16$1$2$1$0$1.000000e-01$-1000$-1000$1000$#  NSignals=6  IDPort=off  TimestampPort=off  ErrorPort=off  RemotePort=off  LengthPort=off  StatusPort=off  StartBits=str2num('[int32(36);int32(56);int32(48);int32(2);int32(0);int32(20)]')  SignalSizes=str2num('[int32(12);int32(8);int32(8);int32(18);int32(2);int32(16)]')  ByteOrders=str2num('[int32(1);int32(1);int32(1);int32(1);int32(1);int32(1)]')  DataTypes=str2num('[int32(2);int32(2);int32(2);int32(2);int32(2);int32(2)]')  MultiplexTypes=str2num('[int32(1);int32(1);int32(1);int32(1);int32(1);int32(1)]')  MultiplexValues=str2num('[double(0);double(0);double(0);double(0);double(0);double(0)]')  Factors=str2num('[double(1);double(1);double(1);double(1.000000e-01);double(1);double(1.000000e-01)]')  Offsets=str2num('[double(-500);double(0);double(-50);double(-10000);double(0);double(-1000)]')  Minimums=str2num('[double(-500);double(0);double(-50);double(-10000);double(0);double(-1000)]')  Maximums=str2num('[double(500);double(255);double(205);double(10000);double(3);double(1000)]')
      settings: DataFormat=CANdb specified signals
  Memory : Memory  InheritSampleTime=on
  Sum : Sum  Inputs=|++  OutDataTypeStr=uint8
  Terminator{1..4} (4 alike) : Terminator
  RR_RPM_Feedback : Outport
  FL_Torque_Feedback : Outport  Port=2
  RL_MotorStatus : Outport  Port=3
  wires:
  Memory/1 -> Sum/2
  Sum/1 -> Memory/1, RL_MotorStatus/1
  Constant/1 -> Sum/1
  msg/1 -> MCU_RR/1
  MCU_RR/1 -> Terminator3/1
  MCU_RR/2 -> Terminator1/1
  MCU_RR/3 -> Terminator2/1
  MCU_RR/4 -> RR_RPM_Feedback/1
  MCU_RR/5 -> Terminator4/1
  MCU_RR/6 -> FL_Torque_Feedback/1

== system w31_v6/CAN_Receive_10ms/Chassis_CAN/RR_Motor_NoMsg ==
  note: 输出1表示信号丢失
      | 输出0表示一切正常
  RxMsgCnt : Inport
  NoRxMsgCntMax : Inport  Port=2
  Chart : Stateflow chart  TreatAsAtomicUnit=on
  Relational Operator1 : RelationalOperator  Operator=~=  OutDataTypeStr=boolean
  Terminator : Terminator
  Unit Delay1 : UnitDelay  SampleTime=-1
  NoRxMsgComfirm : Outport
  wires:
  NoRxMsgCntMax/1 -> Chart/2(NoRxMsgCntMax)
  Unit Delay1/1 -> Relational Operator1/1
  RxMsgCnt/1 -> Relational Operator1/2, Unit Delay1/1
  Relational Operator1/1 -> Chart/1(RxMsg)
  Chart/1(NoRxMsgComfirm) -> NoRxMsgComfirm/1
  Chart/2(NoRxMsgCnt) -> Terminator/1

== system w31_v6/CAN_Receive_10ms/Hardware_Input/DI signal jittered ==
  Key_Ignation : Inport
  Emergency_Stop : Inport  Port=2
  Front_Touch_Switch : Inport  Port=3
  Rear_Touch_Switch : Inport  Port=4
  DI HS signal jitter1 : Subsystem
  DI HS signal jitter2 : Subsystem
  DI HS signal jitter3 : Subsystem
  DI HS signal jitter8 : Subsystem
  Key_In_Cmd : Outport
  Eme_Stop_Cmd : Outport  Port=2
  Front_Touch_Enable : Outport  Port=3
  Rear_Touch_Enable : Outport  Port=4
  wires:
  Key_Ignation/1 -> DI HS signal jitter8/1(DISig)
  DI HS signal jitter8/1(DISigJittered) -> Key_In_Cmd/1
  Emergency_Stop/1 -> DI HS signal jitter1/1(DISig)
  DI HS signal jitter1/1(DISigJittered) -> Eme_Stop_Cmd/1
  Front_Touch_Switch/1 -> DI HS signal jitter3/1(DISig)
  DI HS signal jitter3/1(DISigJittered) -> Front_Touch_Enable/1
  Rear_Touch_Switch/1 -> DI HS signal jitter2/1(DISig)
  DI HS signal jitter2/1(DISigJittered) -> Rear_Touch_Enable/1

== system w31_v6/CAN_Receive_10ms/Hardware_Input/Hardware ==
  note: 52、73引脚反的
  Bus Creator : BusCreator
  Emergency_Stop : iohwablib/DI  text_resource=DI2SG  ts=-1  ECU=V11P51_00E170701_01
  Front_Touch_Switch : iohwablib/DI  text_resource=DI1SG  ts=-1  ECU=V11P51_00E170701_01
  Key_Ignation : iohwablib/DI  text_resource=KeyIgn  ts=-1  ECU=V11P51_00E170701_01
  Rear_Touch_Switch : iohwablib/DI  text_resource=DI3SG  ts=-1  ECU=V11P51_00E170701_01
  Hardware_input : Outport
  wires:
  Bus Creator/1 -> Hardware_input/1  "Hardware_input"
  Key_Ignation/1 -> Bus Creator/1  "Key_Ignation"
  Emergency_Stop/1 -> Bus Creator/2  "Emergency_Stop"
  Front_Touch_Switch/1 -> Bus Creator/3  "Front_Touch_Switch"
  Rear_Touch_Switch/1 -> Bus Creator/4  "Rear_Touch_Switch"

== system w31_v6/CAN_Receive_10ms/Remote_Control_CAN/Remote_IO_situation1 ==
  RxMsgCnt : Inport
  NoRxMsgCntMax : Inport  Port=2
  Chart : Stateflow chart  TreatAsAtomicUnit=on
  Relational Operator1 : RelationalOperator  Operator=~=  OutDataTypeStr=boolean
  Terminator : Terminator
  Unit Delay1 : UnitDelay  SampleTime=-1
  NoRxMsgComfirm : Outport
  wires:
  NoRxMsgCntMax/1 -> Chart/2(NoRxMsgCntMax)
  Unit Delay1/1 -> Relational Operator1/1
  RxMsgCnt/1 -> Relational Operator1/2, Unit Delay1/1
  Relational Operator1/1 -> Chart/1(RxMsg)
  Chart/1(NoRxMsgComfirm) -> NoRxMsgComfirm/1
  Chart/2(NoRxMsgCnt) -> Terminator/1

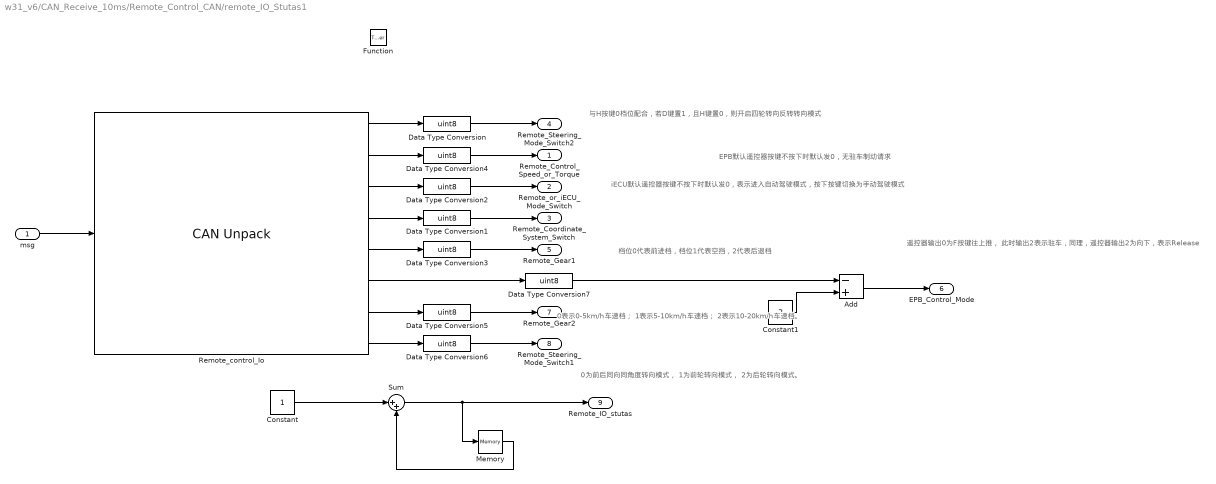
== system w31_v6/CAN_Receive_10ms/Remote_Control_CAN/remote_IO_Stutas1 ==
  note: EPB默认遥控器按键不按下时默认发0，无驻车制动请求
  note: iECU默认遥控器按键不按下时默认发0，表示进入自动驾驶模式，按下按键切换为手动驾驶模式
  note: 档位0代表前进档，档位1代表空挡，2代表后退档
  note: 0表示0-5km/h车速档；
      | 1表示5-10km/h车速档；
      | 2表示10-20km/h车速档。
  note: 0为前后同向同角度转向模式，
      | 1为前轮转向模式，
      | 2为后轮转向模式。
  note: 与H按键0档位配合，若D键置1，且H键置0，则开启四轮转向反转转向模式
  note: 遥控器输出0为F按键往上推，
      | 此时输出2表示驻车，同理，遥控器输出2为向下，表示Release
  msg : Inport
  Function : TriggerPort  TriggerType=function-call  PortDimensions=1
  Add : Sum  Inputs=-+  AccumDataTypeStr=uint8
  Constant : Constant  OutDataTypeStr=uint8  SampleTime=-1
  Constant1 : Constant  Value=2  OutDataTypeStr=uint8  SampleTime=-1
  Data Type Conversion{,1..7} (8 alike) : DataTypeConversion  OutDataTypeStr=uint8
  Memory : Memory  InheritSampleTime=on
  Remote_control_Io : canmsglib/CAN Unpack  CANdbFile=E:\matlab_ws\2012_Matlab_Vcu\w_serial\w3\w32\dbc\w32_CAN1_500kbs_0312_v6.dbc  MsgList=(none)  MsgName=Remote_Control_IO  MsgIDType=Standard (11-bit identifier)  MsgIdentifier=266  MsgLength=8  SignalInfo=Remote_D_Steering_Mode$56$8$1$2$1$0$1$0$0$2$#Remote_A$32$8$1$1$1$0$1$0$0$2$#Remote_B$40$8$1$2$1$0$1$0$0$2$#Remote_C$48$8$1$2$1$0$1$0$0$1$#Remote_E$0$8$1$2$1$0$1$0$0$2$#Remote_F$24$8$1$1$1$0$1$0$0$2$#Remote_G$8$8$1$2$1$0$1$0$0$2$#Remote_H$16$8$1$2$1$0$1$0$0$2$#  NSignals=8  IDPort=off  TimestampPort=off  ErrorPort=off  RemotePort=off  LengthPort=off  StatusPort=off  StartBits=str2num('[int32(56);int32(32);int32(40);int32(48);int32(0);int32(24);int32(8);int32(16)]')  SignalSizes=str2num('[int32(8);int32(8);int32(8);int32(8);int32(8);int32(8);int32(8);int32(8)]')  ByteOrders=str2num('[int32(1);int32(1);int32(1);int32(1);int32(1);int32(1);int32(1);int32(1)]')  DataTypes=str2num('[int32(2);int32(1);int32(2);int32(2);int32(2);int32(1);int32(2);int32(2)]')  MultiplexTypes=str2num('[int32(1);int32(1);int32(1);int32(1);int32(1);int32(1);int32(1);int32(1)]')  MultiplexValues=str2num('[double(0);double(0);double(0);double(0);double(0);double(0);double(0);double(0)]')  Factors=str2num('[double(1);double(1);double(1);double(1);double(1);double(1);double(1);double(1)]')  Offsets=str2num('[double(0);double(0);double(0);double(0);double(0);double(0);double(0);double(0)]')  Minimums=str2num('[double(0);double(0);double(0);double(0);double(0);double(0);double(0);double(0)]')  Maximums=str2num('[double(2);double(2);double(2);double(1);double(2);double(2);double(2);double(2)]')
  Sum : Sum  Inputs=|++  OutDataTypeStr=uint8
  Remote_Control_Speed_or_Torque : Outport
  Remote_or_iECU_Mode_Switch : Outport  Port=2
  Remote_Coordinate_System_Switch : Outport  Port=3
  Remote_Steering_Mode_Switch2 : Outport  Port=4
  Remote_Gear1 : Outport  Port=5
  EPB_Control_Mode : Outport  Port=6
  Remote_Gear2 : Outport  Port=7
  Remote_Steering_Mode_Switch1 : Outport  Port=8
  Remote_IO_stutas : Outport  Port=9
  wires:
  Memory/1 -> Sum/2
  Sum/1 -> Memory/1, Remote_IO_stutas/1
  Constant/1 -> Sum/1
  msg/1 -> Remote_control_Io/1
  Remote_control_Io/1 -> Data Type Conversion/1
  Remote_control_Io/5 -> Data Type Conversion3/1
  Remote_control_Io/6 -> Data Type Conversion7/1
  Remote_control_Io/7 -> Data Type Conversion5/1
  Remote_control_Io/8 -> Data Type Conversion6/1
  Data Type Conversion/1 -> Remote_Steering_Mode_Switch2/1
  Data Type Conversion3/1 -> Remote_Gear1/1
  Data Type Conversion5/1 -> Remote_Gear2/1
  Data Type Conversion6/1 -> Remote_Steering_Mode_Switch1/1
  Remote_control_Io/2 -> Data Type Conversion4/1
  Remote_control_Io/4 -> Data Type Conversion1/1
  Data Type Conversion1/1 -> Remote_Coordinate_System_Switch/1
  Data Type Conversion4/1 -> Remote_Control_Speed_or_Torque/1
  Remote_control_Io/3 -> Data Type Conversion2/1
  Data Type Conversion7/1 -> Add/1
  Constant1/1 -> Add/2
  Add/1 -> EPB_Control_Mode/1
  Data Type Conversion2/1 -> Remote_or_iECU_Mode_Switch/1
